simulink model "GFLIB_Hyst_BAM"  (Simulink 9.3)
settings: Solver=VariableStepAuto  StartTime=0.0  StopTime=10.0  RelTol=1e-3
settings Model: Creator=nxa18952  LastModifiedBy=nxa18952
settings DataIOCC: SaveFormat=Dataset  SignalLoggingSaveFormat=Dataset  ReturnWorkspaceOutputs=on
settings OptimizationCC: LifeSpan=auto
settings DebuggingCC: UnderspecifiedInitializationDetection=Simplified  MergeDetectMultiDrivingBlocksExec=error  FcnCallInpInsideContextMsg=error  SFUnexpectedBacktrackingDiag=error  SFNoUnconditionalDefaultTransitionDiag=error  SFExecutionAtInitializationDiag=warning  ArithmeticOperatorsInVariantConditions=error
settings HardwareCC: ProdBitPerPointer=64  ProdBitPerSizeT=64  ProdBitPerPtrDiffT=64  ProdLargestAtomicFloat=Float  ProdIntDivRoundTo=Zero  ProdEndianess=LittleEndian  ProdWordSize=64  ProdHWDeviceType=Intel->x86-64 (Windows64)
settings ModelReferenceCC: PropagateSignalLabelsOutOfModel=on
settings SFSimCC: SimUseLocalCustomCode=on
settings RTWCC: RTWUseLocalCustomCode=on
settings CodeAppCC: StateflowObjectComments=off
settings GRTTargetCC: TargetLangStandard=C99 (ISO)  CombineOutputUpdateFcns=on  GRTInterface=off
settings ConfigComp: CovMetricSettings=dwe  CovHtmlReporting=off  CovSaveCumulativeToWorkspaceVar=off  CovSaveSingleToWorkspaceVar=off  CovExternalEMLEnable=on

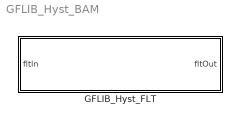
== system GFLIB_Hyst_BAM ==
  GFLIB_Hyst_FLT : Subsystem  TreatAsAtomicUnit=on  mask(GFLIB_Hyst_FLT){showStates=Hide (faster execution), fltHystOn=0, fltHystOff=0, fltOutValOn=0, fltOutValOff=0}
      mask prompts: showStates "Show internal states"; fltHystOn "fltHystOn (Value determining the upper threshold)"; fltHystOff "fltHystOff (Value determining the lower threshold)"; fltOutValOn "fltOutValOn (Value of the output when input is higher than the upper threshold)"; fltOutValOff "fltOutValOff (Value of the output when input is lower than the lower threshold)"
      mask help: Hysteresis function in single precision floating-point implementation. Refer to the AMMCLIB User's Guide for further details.
      mask init:
      | if ~evalin('base','exist(''tS8'',''var'')')
      |   if (2 ~= exist('SWLIBS_Typedefs.mat','file'))
      |       error('File SWLIBS_Typedefs.mat is not on the Matlab path. Please add the AMMCLIB "bam" folder in the Matlab Search Path.');
      |   else
      |       evalin('base', 'load(''SWLIBS_Typedefs.mat'')');
      |   end
      | end
      | if showStates == 1
      |     % hidden state variables
      |     if strcmp(get_param([gcb '/fltHystOn'], 'BlockType'), 'Inport')
      |         posblk = get_param(gcb, 'Position');
      | 
      |         pos = get_param(    [gcb, '/fltHystOn'], 'Position');
      |         orient = get_param( [gcb, '/fltHystOn'], 'Orientation');
      |         delete_block(       [gcb, '/fltHystOn']);
      |         add_block('built-in/Ground', [gcb, '/fltHystOn'], 'Position', pos, 'Orientation', orient);
      | 
      |         pos = get_param(    [gcb, '/fltHystOff'], 'Position');
      |         orient = get_param( [gcb, '/fltHystOff'], 'Orientation');
      |         delete_block(       [gcb, '/fltHystOff']);
      |         add_block('built-in/Ground', [gcb, '/fltHystOff'], 'Position', pos, 'Orientation', orient);
      | 
      |         pos = get_param(    [gcb, '/fltOutValOn'], 'Position');
      |         orient = get_param( [gcb, '/fltOutValOn'], 'Orientation');
      |         delete_block(       [gcb, '/fltOutValOn']);
      |         add_block('built-in/Ground', [gcb, '/fltOutValOn'], 'Position', pos, 'Orientation', orient);
      | 
      |         pos = get_param(    [gcb, '/fltOutValOff'], 'Position');
      |         orient = get_param( [gcb, '/fltOutValOff'], 'Orientation');
      |         delete_block(       [gcb, '/fltOutValOff']);
      |         add_block('built-in/Ground', [gcb, '/fltOutValOff'], 'Position', pos, 'Orientation', orient);
      | 
      |         pos = get_param(    [gcb, '/fltOutState'], 'Position');
      |         orient = get_param( [gcb, '/fltOutState'], 'Orientation');
      |         delete_block(       [gcb, '/fltOutState']);
      |         add_block('built-in/Ground', [gcb, '/fltOutState'], 'Position', pos, 'Orientation', orient);
      | 
      | 
      |         pos = get_param(    [gcb '/fltOutState_Out'], 'Position');
      |         orient = get_param( [gcb '/fltOutState_Out'], 'Orientation');
      |         delete_block(       [gcb '/fltOutState_Out']);
      |         add_block('built-in/Terminator', [gcb '/fltOutState_Out'], 'Position', pos, 'Orientation', orient);
      | 
      | 
      |         set_param([gcb '/fltIn'], 'Port', '1');
      | 
      |         set_param([gcb '/fltOut'], 'Port', '1');
      | 
      |         set_param(gcb,'MaskEnables',{'on','on','on','on','on'});
      | 
      |         if (posblk(4) - posblk(2)) > 50
      |           height = 50;
      |           set_param(gcb,'Position',[posblk(1), posblk(2), posblk(3), posblk(2)+height])
      |         end
      |     end
      | else
      |     % shown state variables
      |     if strcmp(get_param([gcb '/fltHystOn'], 'BlockType'), 'Ground')
      |         posblk = get_param(gcb, 'Position');
      | 
      |         pos = get_param(    [gcb, '/fltHystOn'], 'Position');
      |         orient = get_param( [gcb, '/fltHystOn'], 'Orientation');
      |         delete_block(       [gcb, '/fltHystOn']);
      |         add_block('built-in/Inport', [gcb, '/fltHystOn'], 'Position', pos, 'Orientation', orient, 'OutDataTypeStr', 'single');
      | 
      |         pos = get_param(    [gcb, '/fltHystOff'], 'Position');
      |         orient = get_param( [gcb, '/fltHystOff'], 'Orientation');
      |         delete_block(       [gcb, '/fltHystOff']);
      |         add_block('built-in/Inport', [gcb, '/fltHystOff'], 'Position', pos, 'Orientation', orient, 'OutDataTypeStr', 'single');
      | 
      |         pos = get_param(    [gcb, '/fltOutValOn'], 'Position');
      |         orient = get_param( [gcb, '/fltOutValOn'], 'Orientation');
      |         delete_block(       [gcb, '/fltOutValOn']);
      |         add_block('built-in/Inport', [gcb, '/fltOutValOn'], 'Position', pos, 'Orientation', orient, 'OutDataTypeStr', 'single');
      | 
      |         pos = get_param(    [gcb, '/fltOutValOff'], 'Position');
      |         orient = get_param( [gcb, '/fltOutValOff'], 'Orientation');
      |         delete_block(       [gcb, '/fltOutValOff']);
      |         add_block('built-in/Inport', [gcb, '/fltOutValOff'], 'Position', pos, 'Orientation', orient, 'OutDataTypeStr', 'single');
      | 
      |         pos = get_param(    [gcb, '/fltOutState'], 'Position');
      |         orient = get_param( [gcb, '/fltOutState'], 'Orientation');
      |         delete_block(       [gcb, '/fltOutState']);
      |         add_block('built-in/Inport', [gcb, '/fltOutState'], 'Position', pos, 'Orientation', orient, 'OutDataTypeStr', 'single');
      | 
      | 
      |         pos = get_param(    [gcb '/fltOutState_Out'], 'Position');
      |         orient = get_param( [gcb '/fltOutState_Out'], 'Orientation');
      |         delete_block(       [gcb '/fltOutState_Out']);
      |         add_block('built-in/Outport', [gcb '/fltOutState_Out'], 'Position', pos, 'Orientation', orient);
      | 
      | 
      |         set_param([gcb '/fltIn'], 'Port', '1');
      |         set_param([gcb '/fltHystOn'], 'Port', '2');
      |         set_param([gcb '/fltHystOff'], 'Port', '3');
      |         set_param([gcb '/fltOutValOn'], 'Port', '4');
      |         set_param([gcb '/fltOutValOff'], 'Port', '5');
      |         set_param([gcb '/fltOutState'], 'Port', '6');
      | 
      |         set_param([gcb '/fltOut'], 'Port', '1');
      |         set_param([gcb '/fltOutState_Out'], 'Port', '2');
      | 
      |         set_param(gcb,'MaskEnables',{'on','off','off','off','off'});
      | 
      |         if (posblk(4) - posblk(2)) < 175
      |           height = 175;
      |           set_param(gcb,'Position',[posblk(1), posblk(2), posblk(3), posblk(2)+height])
      |         end
      |     end
      | end
      settings: RTWSystemCode=Inline
      mask TypeOptions showStates: Hide (faster execution) | Show (allows debugging; connect feedback loops manually)
      mask Callback showStates:
      | maskStr = get_param(gcb,'showStates');
      | if strcmp(maskStr,'Hide (faster execution)'),
      |     set_param(gcb,'MaskEnables',{'on','on','on','on','on'});
      | else
      |     set_param(gcb,'MaskEnables',{'on','off','off','off','off'});
      | end
      mask Display:
      | color('black');
      | pos = get_param(gcb, 'Position');
      | width = pos(3) - pos(1);
      | height = pos(4) - pos(2);
      | tX=width/2;
      | tY=height - 8;
      | color('black');
      | text(tX,tY, 'GFLIB_Hyst_FLT', 'horizontalAlignment', 'center');
      | if showStates == 2
      |   color('red');
      |   text(tX,tY - 20, ['debugging mode' char(13) char(10) '(limited performance)'], 'horizontalAlignment', 'center');
      | end

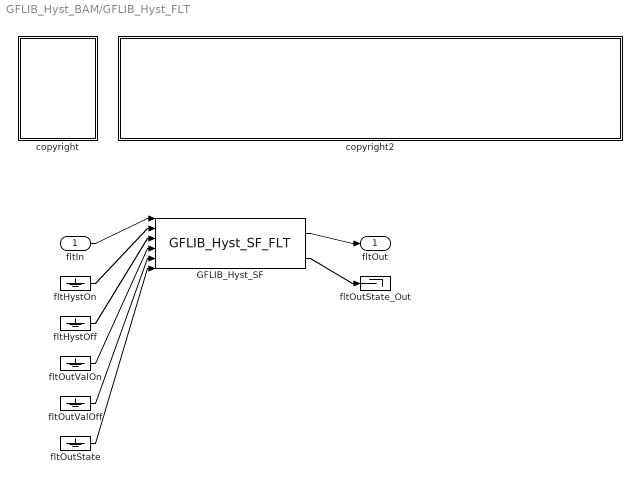
== system GFLIB_Hyst_BAM/GFLIB_Hyst_FLT ==
  fltIn : Inport  OutDataTypeStr=single
  GFLIB_Hyst_SF : S-Function  FunctionName=GFLIB_Hyst_SF_FLT  Parameters=showStates,fltHystOn,fltHystOff,fltOutValOn,fltOutValOff  SFunctionDeploymentMode=off  EnableBusSupport=off
  copyright : Subsystem
      mask Display: text(10,90,'FILE:');text(10,75,'DESRIPTION:');text(10,60,'COPYRIGHT:');text(10,45,'VERSION:');text(10,30,'DATE:')
  copyright2 : Subsystem
      mask Display: text(10,90,'GFLIB_Hyst_BAM_FLT.mdl');text(10,75,'Hysteresis function.');text(10,60,'NXP 2020');text(10,45,'1.0');text(10,30,'18-Mar-2020');
  fltHystOff : Ground
  fltHystOn : Ground
  fltOutState : Ground
  fltOutState_Out : Terminator
  fltOutValOff : Ground
  fltOutValOn : Ground
  fltOut : Outport
  wires:
  fltIn/1 -> GFLIB_Hyst_SF/1
  fltHystOn/1 -> GFLIB_Hyst_SF/2
  fltHystOff/1 -> GFLIB_Hyst_SF/3
  fltOutValOn/1 -> GFLIB_Hyst_SF/4
  fltOutValOff/1 -> GFLIB_Hyst_SF/5
  fltOutState/1 -> GFLIB_Hyst_SF/6
  GFLIB_Hyst_SF/1 -> fltOut/1
  GFLIB_Hyst_SF/2 -> fltOutState_Out/1

== system GFLIB_Hyst_BAM/GFLIB_Hyst_FLT/copyright ==

== system GFLIB_Hyst_BAM/GFLIB_Hyst_FLT/copyright2 ==
